simulink model "projectnckh"  (R2018a)
settings: Solver=ode45  StartTime=0.0  StopTime=10  RelTol=1e-3
values from neighbouring files (symbols this model uses):
  L = 12    [Run_mohinh1_2.m]
  M = 4200    [Run_mohinh1_2.m]
undefined symbols (not defined in the file or in its folder): C1, C2, CL1, CL2, hg, K1, K2, KL1, KL2, m1, M1, m2, M2, M3, q0, S, sigbuilder_block, t4, V
settings Model: Creator=admin  LastModifiedBy=admin
settings SolverCC: AlgebraicLoopSolver=LineSearch

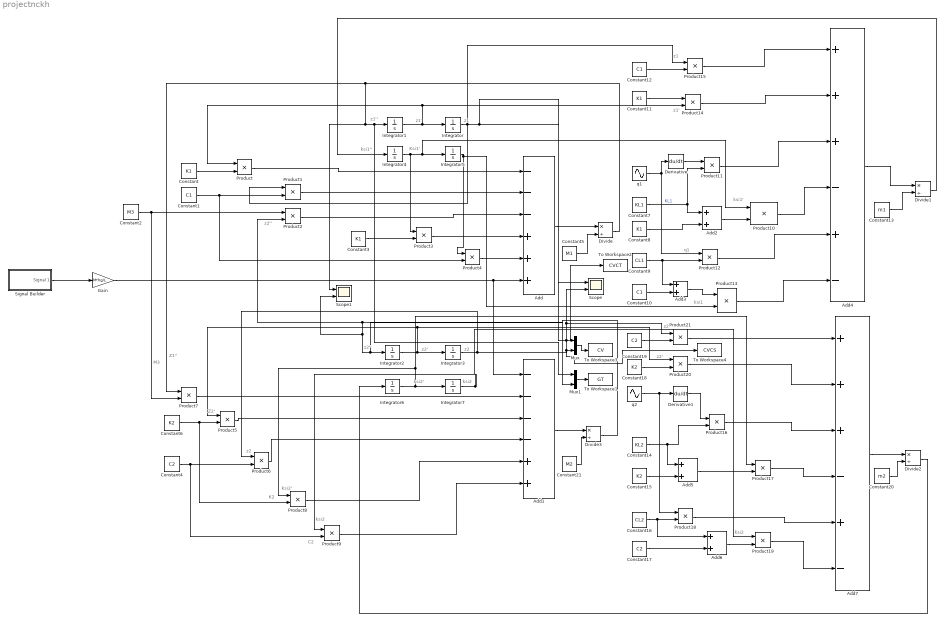
== system projectnckh ==
  note: z2
  note: z2'
  note: ksi2
  note: ksi1''
  note: q1
  note: z1'
  note: ksi1
  note: ksi1'
  note: z2''
  note: z2''
  note: C2
  note: ksi2
  note: ksi2
  note: ksi2'
  note: K2
  note: z2
  note: Z2'
  note: ksi2'
  note: Z1''
  note: M3
  note: z2
  note: z2'
  note: z1''
  note: Ksi1'
  note: z1
  note: z1'
  note: z1
  Add : Sum  Inputs=---+++
  Add1 : Sum  Inputs=----++
  Add{2..3,5..6} (4 alike) : Sum
  Add4 : Sum  Inputs=+++-+-
  Add7 : Sum  Inputs=+++-+-
  Constant{,3,8,11} (4 alike) : Constant  Value=K1
  Constant1 : Constant  Value=C1
  Constant10 : Constant  Value=C1
  Constant12 : Constant  Value=C1
  Constant13 : Constant  Value=m1
  Constant14 : Constant  Value=KL2
  Constant15 : Constant  Value=K2
  Constant16 : Constant  Value=CL2
  Constant17 : Constant  Value=C2
  Constant18 : Constant  Value=K2
  Constant19 : Constant  Value=C2
  Constant2 : Constant  Value=M3
  Constant20 : Constant  Value=m2
  Constant21 : Constant  Value=M2
  Constant4 : Constant  Value=C2
  Constant5 : Constant  Value=M1
  Constant6 : Constant  Value=K2
  Constant7 : Constant  Value=KL1
  Constant9 : Constant  Value=CL1
  Derivative : Derivative
  Derivative1 : Derivative
  Divide{,1..3} (4 alike) : Product  Inputs=*/
  Gain : Gain  Gain=M*hg/L
  Integrator{,1..7} (8 alike) : Integrator
  Mux : Mux  Inputs=2
  Mux1 : Mux  Inputs=2
  Product{,1..21} (22 alike) : Product
  Scope : Scope  NumInputPorts=2
  Scope1 : Scope  NumInputPorts=2
  Signal Builder : Subsystem  Tag=STV Subsys  LoadFcn=sigbuilder_block('load');  StartFcn=sigbuilder_block('start');  StopFcn=sigbuilder_block('stop');  ClipboardFcn=sigbuilder_block('clipboard');  mask(Sigbuilder block){tuvar=[0:10]}
      mask help: Simulink:masks:SigbuilderBlock_MD
      mask init:
      | if ~strcmp(get_param(bdroot(gcbh),'SimulationStatus'),'stopped') tuvar = sigbuilder_block('maskInit'); end
      settings: CopyFcn=sigbuilder_block('copy');  DeleteFcn=sigbuilder_block('delete');  ModelCloseFcn=sigbuilder_block('modelClose');  PreSaveFcn=sigbuilder_block('preSave');  PauseFcn=sigbuilder_block('pause');  ContinueFcn=sigbuilder_block('continue');  NameChangeFcn=sigbuilder_block('namechange');  OpenFcn=sigbuilder_block('open',[436.8 165 550.8 400.2 ]);  CloseFcn=sigbuilder_block('close');
      mask Display: plot(0, 0, 100, 100,[2, 2, 32, 32, 2], [68, 8, 8, 68, 68],[32, 2], [38, 38], [32, 19, 2],[53, 60, 44], [32, 17, 17, 2],[16, 16, 31, 31]);txt = getActiveGroup(gcbh);text(2, 100, txt,'verticalAlignment', 'top');
  To Workspace1 : ToWorkspace  VariableName=GT  SaveFormat=Timeseries  SampleTime=-1
  To Workspace2 : ToWorkspace  VariableName=CVCT  SaveFormat=Timeseries  SampleTime=-1
  To Workspace3 : ToWorkspace  VariableName=CV  SaveFormat=Timeseries  SampleTime=-1
  To Workspace4 : ToWorkspace  VariableName=CVCS  SaveFormat=Timeseries  SampleTime=-1
  q1 : Sin  TimeSource=Use external signal  Amplitude=q0  Frequency=(2*pi*V)/S  SampleTime=0
  q2 : Sin  TimeSource=Use external signal  Amplitude=q0  Frequency=(2*pi*V)/S  Phase=-(2*pi*t4*V)/S  SampleTime=0
  wires:
  Integrator1/1 -> Product14/2, Product/1, Integrator/1
  Signal Builder/1(Signal 1) -> Gain/1
  Constant/1 -> Product/2
  Integrator2/1 -> Product20/1, Product5/1, Integrator3/1
  Integrator4/1 -> Product3/1, Product10/1, Integrator5/1
  Constant2/1 -> Product2/1, Product7/2
  Constant3/1 -> Product3/2
  Constant1/1 -> Product4/2, Product1/2
  Integrator5/1 -> Product13/2, Product4/1
  Product/1 -> Add/1
  Product1/1 -> Add/2
  Product2/1 -> Add/3
  Product3/1 -> Add/4
  Product4/1 -> Add/5
  Gain/1 -> Add1/1, Add/6
  Add/1 -> Divide/1
  Constant5/1 -> Divide/2
  Divide/1 -> Product7/1, Scope1/1, Mux1/1, Integrator1/1
  Constant6/1 -> Product8/2, Product5/2
  Constant4/1 -> Product9/2, Product6/2
  Integrator6/1 -> Product17/1, Product8/1, Integrator7/1
  Product7/1 -> Add1/2
  Product5/1 -> Add1/3
  Product6/1 -> Add1/4
  Product8/1 -> Add1/5
  Product9/1 -> Add1/6
  Divide3/1 -> Scope1/2, Mux1/2, Integrator2/1, Product2/2
  Constant7/1 -> Add2/1, Product11/2  "KL1"
  Constant8/1 -> Add2/2
  Add2/1 -> Product10/2
  q1/1 -> Product12/1, Derivative/1
  Derivative/1 -> Product11/1
  Constant9/1 -> Add3/1, Product12/2
  Constant10/1 -> Add3/2
  Add3/1 -> Product13/1
  Constant11/1 -> Product14/1
  Constant12/1 -> Product15/2
  Product15/1 -> Add4/1
  Product14/1 -> Add4/2
  Product11/1 -> Add4/3
  Product10/1 -> Add4/4
  Product12/1 -> Add4/5
  Product13/1 -> Add4/6
  Add4/1 -> Divide1/1
  Constant13/1 -> Divide1/2
  Divide1/1 -> Integrator4/1
  q2/1 -> Product18/1, Derivative1/1
  Derivative1/1 -> Product16/1
  Constant14/1 -> Add5/1, Product16/2
  Constant15/1 -> Add5/2
  Add5/1 -> Product17/2
  Constant16/1 -> Add6/1, Product18/2
  Constant17/1 -> Add6/2
  Add6/1 -> Product19/2
  Integrator7/1 -> Product19/1, Product9/1
  Constant18/1 -> Product20/2
  Constant19/1 -> Product21/2
  Product21/1 -> Add7/1
  Product20/1 -> Add7/2
  Product16/1 -> Add7/3
  Product17/1 -> Add7/4
  Product18/1 -> Add7/5
  Product19/1 -> Add7/6
  Add7/1 -> Divide2/1
  Constant20/1 -> Divide2/2
  Divide2/1 -> Integrator6/1
  Integrator3/1 -> To Workspace4/1, Mux/2, Scope/2, Product21/1, Product6/1
  Integrator/1 -> To Workspace2/1, Mux/1, Scope/1, Product15/1, Product1/1
  Constant21/1 -> Divide3/2
  Add1/1 -> Divide3/1
  Mux/1 -> To Workspace3/1
  Mux1/1 -> To Workspace1/1

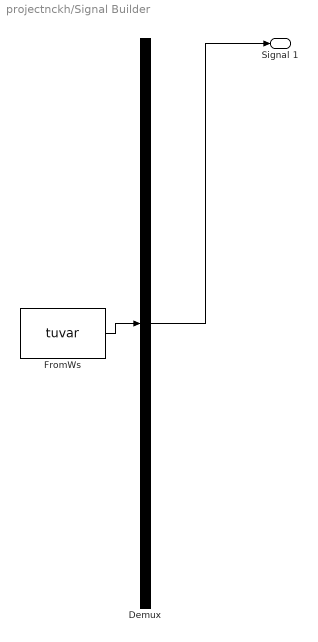
== system projectnckh/Signal Builder ==
  Demux : Demux  Tag=STV Demux  Outputs=1
  FromWs : FromWorkspace  Tag=STV FromWs  VariableName=tuvar  SampleTime=0
      SigBuilderData=|
      | common.afterFinalStr = 'Extrapolate'
      | common.sampleTime = 0
      | dataSet.timeRange = [0 7]
      | dataSet.name = 'Group 1'
      | sbobj.Groups.Name = 'Group 1'
      | sbobj.Groups.Signals.Name = 'Signal 1'
      | sbobj.Groups.Signals.XData = [0 0.6 0.65 2.514 2.714 7]
      | sbobj.Groups.Signals.YData = [0 0 6 6 0 0]
      | sbobj.Groups.TimeRange = [0 7]
  Signal 1 : Outport  Tag=STV Outport
  wires:
  Demux/1 -> Signal 1/1
  FromWs/1 -> Demux/1
